simulink model "momentum_controller"  (R2020b)
settings: Solver=VariableStepAuto  StartTime=0.0  StopTime=100  RelTol=1e-3
values from neighbouring files (symbols this model uses):
  J = 0.001    [PMSM_params.m]
  Ls = 0.1    [PMSM_params.m]
  Lsd = Ls    (= 0.1)    [PMSM_params.m]
  Lsq = Ls    (= 0.1)    [PMSM_params.m]
  psi_f = 1    [PMSM_params.m]
  Rs = 10    [PMSM_params.m]
  Z = 1    [PMSM_params.m]
libraries: pid_lib x2
settings Model: Creator=Алексей  LastModifiedBy=Алексей

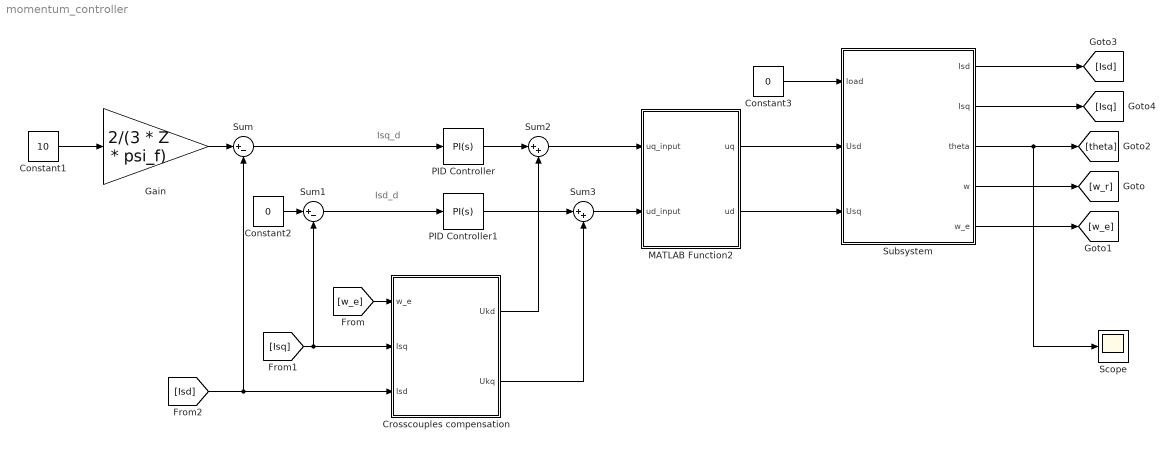
== system momentum_controller ==
  note: Isd_d
  note: Isq_d
  Constant1 : Constant  Value=10
  Constant2 : Constant  Value=0
  Constant3 : Constant  Value=0
  Crosscouples compensation : Subsystem
  Gain : Gain  Gain=2/(3 * Z * psi_f)
  MATLAB Function2 : MATLAB Function  TreatAsAtomicUnit=on
  PID Controller : pid_lib/PID Controller  Controller=PI  Form=Parallel  TimeDomain=Continuous-time  UseExternalTs=off  SampleTime=-1  IntegratorMethod=Forward Euler  FilterMethod=Forward Euler  ControllerParametersSource=internal  P=1  I=1  D=0  UseFilter=on  N=100  TunerSelectOption=Transfer Function Based (PID Tuner App)  InitialConditionSource=internal  InitialConditionForIntegrator=0  InitialConditionForFilter=0  DifferentiatorICPrevScaledInput=0  ExternalReset=none  TrackingMode=off  Kt=1  LimitOutput=off  SatLimitsSource=internal  UpperSaturationLimit=inf  LowerSaturationLimit=-inf  LinearizeAsGain=on  AntiWindupMode=none  Kb=1  POutMin=[]  POutMax=[]  IOutMin=[]  IOutMax=[]  DOutMin=[]  DOutMax=[]  NOutMin=[]  NOutMax=[]  SumOutMin=[]  SumOutMax=[]  SaturationOutMin=[]  SaturationOutMax=[]  PParamMin=[]  PParamMax=[]  IParamMin=[]  IParamMax=[]  DParamMin=[]  DParamMax=[]  NParamMin=[]  NParamMax=[]  KbParamMin=[]  KbParamMax=[]  KtParamMin=[]  KtParamMax=[]  KbOutMin=[]  KbOutMax=[]  KtOutMin=[]  KtOutMax=[]  IntegratorOutMin=[]  IntegratorOutMax=[]  FilterOutMin=[]  FilterOutMax=[]  SumI1OutMin=[]  SumI1OutMax=[]  SumI2OutMin=[]  SumI2OutMax=[]  SumI3OutMin=[]  SumI3OutMax=[]  SumI4OutMin=[]  SumI4OutMax=[]  SumDOutMin=[]  SumDOutMax=[]  DifferentiatorOutMin=[]  DifferentiatorOutMax=[]  FilterDiffOutCoefMin=[]  FilterDiffOutCoefMax=[]  ReciprocalOutMin=[]  ReciprocalOutMax=[]  SumDenOutMin=[]  SumDenOutMax=[]  SumNumOutMin=[]  SumNumOutMax=[]  DivideOutMin=[]  DivideOutMax=[]  UdiffTsProdOutMin=[]  UdiffTsProdOutMax=[]  NTsProdOutMin=[]  NTsProdOutMax=[]  UintegralTsProdOutMin=[]  UintegralTsProdOutMax=[]  UngainTsProdOutMin=[]  UngainTsProdOutMax=[]  IntegratorContinuousStateAttributes=''  IntegratorStateMustResolveToSignalObject=off  IntegratorRTWStateStorageClass=Auto  FilterContinuousStateAttributes=''  FilterStateMustResolveToSignalObject=off  FilterRTWStateStorageClass=Auto  ParallelPVariant=InternalParameters  IdealPVariant=Disabled  IVariant=InternalParameters  DVariant=Disabled  IntegratorVariant=Continuous  SatVariant=Disabled  AWVariant=Passthrough  PCopyVariant=Disabled  TRVariant=Disabled  FdbkBlocksVariant=Forward  IdealPFdbkVariant=Disabled  SatFdbkVariant=Disabled  DerivativeFilterVariant=Disabled  NVariant=Disabled  NCopyVariant=Disabled_SignalSpec  FilterICVariant=Disabled  IntegratorICVariant=InternalICs  ExternalResetVariant=Disabled  TRSumVariant=Passthrough  SumFdbkVariant=Disabled  SumVariant=Sum_PI  TsampFilterVariant=InternalTs  TsampNgainVariant=Passthrough  TsampIntegralVariant=Passthrough  ExternalSaturationOutDataTypeStr=Inherit: Same as second input
  PID Controller1 : pid_lib/PID Controller  Controller=PI  Form=Parallel  TimeDomain=Continuous-time  UseExternalTs=off  SampleTime=-1  IntegratorMethod=Forward Euler  FilterMethod=Forward Euler  ControllerParametersSource=internal  P=1  I=1  D=0  UseFilter=on  N=100  TunerSelectOption=Transfer Function Based (PID Tuner App)  InitialConditionSource=internal  InitialConditionForIntegrator=0  InitialConditionForFilter=0  DifferentiatorICPrevScaledInput=0  ExternalReset=none  TrackingMode=off  Kt=1  LimitOutput=off  SatLimitsSource=internal  UpperSaturationLimit=inf  LowerSaturationLimit=-inf  LinearizeAsGain=on  AntiWindupMode=none  Kb=1  POutMin=[]  POutMax=[]  IOutMin=[]  IOutMax=[]  DOutMin=[]  DOutMax=[]  NOutMin=[]  NOutMax=[]  SumOutMin=[]  SumOutMax=[]  SaturationOutMin=[]  SaturationOutMax=[]  PParamMin=[]  PParamMax=[]  IParamMin=[]  IParamMax=[]  DParamMin=[]  DParamMax=[]  NParamMin=[]  NParamMax=[]  KbParamMin=[]  KbParamMax=[]  KtParamMin=[]  KtParamMax=[]  KbOutMin=[]  KbOutMax=[]  KtOutMin=[]  KtOutMax=[]  IntegratorOutMin=[]  IntegratorOutMax=[]  FilterOutMin=[]  FilterOutMax=[]  SumI1OutMin=[]  SumI1OutMax=[]  SumI2OutMin=[]  SumI2OutMax=[]  SumI3OutMin=[]  SumI3OutMax=[]  SumI4OutMin=[]  SumI4OutMax=[]  SumDOutMin=[]  SumDOutMax=[]  DifferentiatorOutMin=[]  DifferentiatorOutMax=[]  FilterDiffOutCoefMin=[]  FilterDiffOutCoefMax=[]  ReciprocalOutMin=[]  ReciprocalOutMax=[]  SumDenOutMin=[]  SumDenOutMax=[]  SumNumOutMin=[]  SumNumOutMax=[]  DivideOutMin=[]  DivideOutMax=[]  UdiffTsProdOutMin=[]  UdiffTsProdOutMax=[]  NTsProdOutMin=[]  NTsProdOutMax=[]  UintegralTsProdOutMin=[]  UintegralTsProdOutMax=[]  UngainTsProdOutMin=[]  UngainTsProdOutMax=[]  IntegratorContinuousStateAttributes=''  IntegratorStateMustResolveToSignalObject=off  IntegratorRTWStateStorageClass=Auto  FilterContinuousStateAttributes=''  FilterStateMustResolveToSignalObject=off  FilterRTWStateStorageClass=Auto  ParallelPVariant=InternalParameters  IdealPVariant=Disabled  IVariant=InternalParameters  DVariant=Disabled  IntegratorVariant=Continuous  SatVariant=Disabled  AWVariant=Passthrough  PCopyVariant=Disabled  TRVariant=Disabled  FdbkBlocksVariant=Forward  IdealPFdbkVariant=Disabled  SatFdbkVariant=Disabled  DerivativeFilterVariant=Disabled  NVariant=Disabled  NCopyVariant=Disabled_SignalSpec  FilterICVariant=Disabled  IntegratorICVariant=InternalICs  ExternalResetVariant=Disabled  TRSumVariant=Passthrough  SumFdbkVariant=Disabled  SumVariant=Sum_PI  TsampFilterVariant=InternalTs  TsampNgainVariant=Passthrough  TsampIntegralVariant=Passthrough  ExternalSaturationOutDataTypeStr=Inherit: Same as second input
  Scope : Scope
  Subsystem : Subsystem
  Sum : Sum  Inputs=|+-
  Sum1 : Sum  Inputs=|+-
  Sum2 : Sum  Inputs=|++
  Sum3 : Sum  Inputs=|++
  wires:
  Constant1/1 -> Gain/1
  Gain/1 -> Sum/1
  Sum/1 -> PID Controller/1
  Constant2/1 -> Sum1/1
  Sum1/1 -> PID Controller1/1
  Constant3/1 -> Subsystem/1(load)
  Subsystem/3(theta) -> Scope/1, [theta]
  Subsystem/4(w) -> [w_r]
  Subsystem/5(w_e) -> [w_e]
  Subsystem/2(Isq) -> [Isq]
  Subsystem/1(Isd) -> [Isd]
  [w_e] -> Crosscouples compensation/1(w_e)
  [Isq] -> Sum1/2, Crosscouples compensation/2(Isq)
  [Isd] -> Crosscouples compensation/3(Isd), Sum/2
  PID Controller1/1 -> Sum3/1
  PID Controller/1 -> Sum2/1
  Crosscouples compensation/1(Ukd) -> Sum2/2
  Crosscouples compensation/2(Ukq) -> Sum3/2
  MATLAB Function2/1(uq) -> Subsystem/2(Usd)
  MATLAB Function2/2(ud) -> Subsystem/3(Usq)
  Sum2/1 -> MATLAB Function2/1(uq_input)
  Sum3/1 -> MATLAB Function2/2(ud_input)

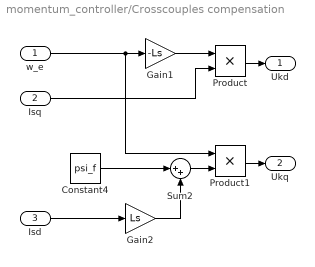
== system momentum_controller/Crosscouples compensation ==
  w_e : Inport
  Isq : Inport  Port=2
  Isd : Inport  Port=3
  Constant4 : Constant  Value=psi_f
  Gain1 : Gain  Gain=-Ls
  Gain2 : Gain  Gain=Ls
  Product : Product
  Product1 : Product
  Sum2 : Sum  Inputs=|++
  Ukd : Outport
  Ukq : Outport  Port=2
  wires:
  Isq/1 -> Product/2
  Gain2/1 -> Sum2/2
  w_e/1 -> Product1/1, Gain1/1
  Product/1 -> Ukd/1
  Constant4/1 -> Sum2/1
  Gain1/1 -> Product/1
  Product1/1 -> Ukq/1
  Isd/1 -> Gain2/1
  Sum2/1 -> Product1/2

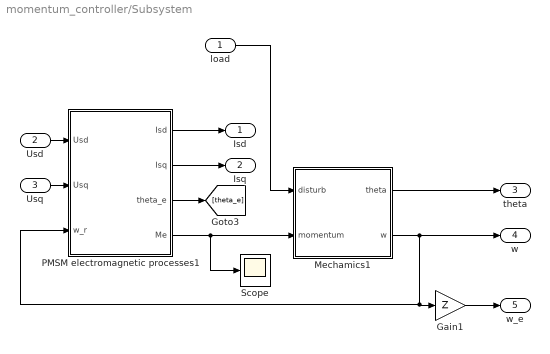
== system momentum_controller/Subsystem ==
  load : Inport
  Usd : Inport  Port=2
  Usq : Inport  Port=3
  Gain1 : Gain  Gain=Z
  Mechamics1 : Subsystem
  PMSM electromagnetic processes1 : Subsystem
  Scope : Scope
  Isd : Outport
  Isq : Outport  Port=2
  theta : Outport  Port=3
  w : Outport  Port=4
  w_e : Outport  Port=5
  wires:
  Mechamics1/2(w) -> w/1, PMSM electromagnetic processes1/3(w_r), Gain1/1
  PMSM electromagnetic processes1/3(theta_e) -> [theta_e]
  PMSM electromagnetic processes1/4(Me) -> Scope/1, Mechamics1/2(momentum)
  PMSM electromagnetic processes1/1(Isd) -> Isd/1
  Mechamics1/1(theta) -> theta/1
  Gain1/1 -> w_e/1
  load/1 -> Mechamics1/1(disturb)
  Usd/1 -> PMSM electromagnetic processes1/1(Usd)
  Usq/1 -> PMSM electromagnetic processes1/2(Usq)
  PMSM electromagnetic processes1/2(Isq) -> Isq/1

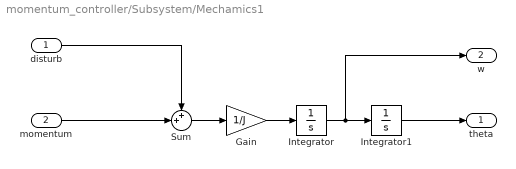
== system momentum_controller/Subsystem/Mechamics1 ==
  disturb : Inport
  momentum : Inport  Port=2
  Gain : Gain  Gain=1/J
  Integrator : Integrator
  Integrator1 : Integrator
  Sum : Sum  Inputs=++|
  theta : Outport  VectorParamsAs1DForOutWhenUnconnected=off
  w : Outport  Port=2  VectorParamsAs1DForOutWhenUnconnected=off
  wires:
  Gain/1 -> Integrator/1
  Sum/1 -> Gain/1
  Integrator1/1 -> theta/1
  momentum/1 -> Sum/2
  disturb/1 -> Sum/1
  Integrator/1 -> Integrator1/1, w/1

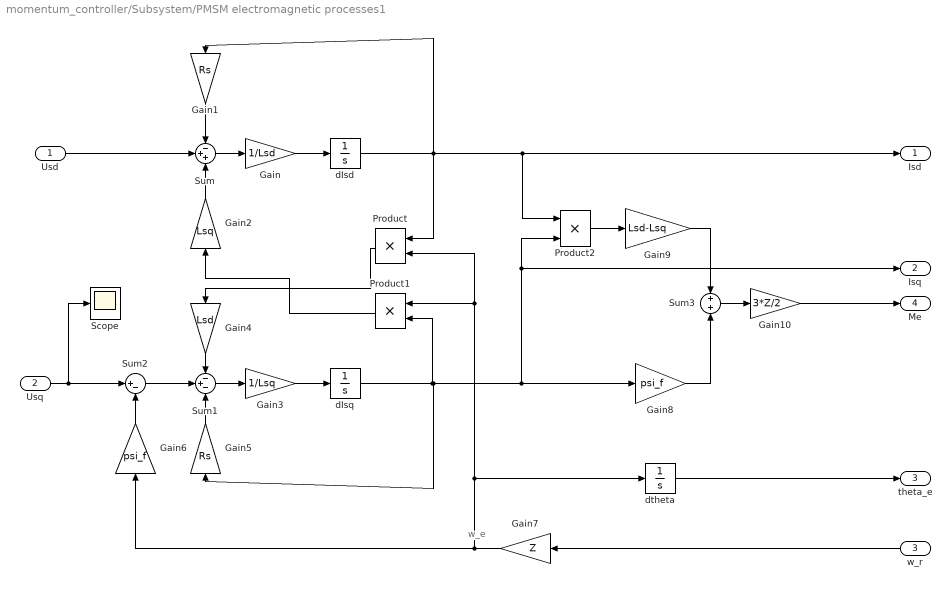
== system momentum_controller/Subsystem/PMSM electromagnetic processes1 ==
  note: w_e
  Usd : Inport
  Usq : Inport  Port=2
  w_r : Inport  Port=3
  Gain : Gain  Gain=1/Lsd
  Gain1 : Gain  Gain=Rs
  Gain10 : Gain  Gain=3*Z/2
  Gain2 : Gain  Gain=Lsq
  Gain3 : Gain  Gain=1/Lsq
  Gain4 : Gain  Gain=Lsd
  Gain5 : Gain  Gain=Rs
  Gain6 : Gain  Gain=psi_f
  Gain7 : Gain  Gain=Z
  Gain8 : Gain  Gain=psi_f
  Gain9 : Gain  Gain=Lsd-Lsq
  Product : Product
  Product1 : Product
  Product2 : Product
  Scope : Scope
  Sum : Sum  Inputs=-++
  Sum1 : Sum  Inputs=-+-
  Sum2 : Sum  Inputs=|+-
  Sum3 : Sum
  dIsd : Integrator
  dIsq : Integrator
  dtheta : Integrator
  Isd : Outport  VectorParamsAs1DForOutWhenUnconnected=off
  Isq : Outport  Port=2  VectorParamsAs1DForOutWhenUnconnected=off
  theta_e : Outport  Port=3  VectorParamsAs1DForOutWhenUnconnected=off
  Me : Outport  Port=4  VectorParamsAs1DForOutWhenUnconnected=off
  wires:
  Gain4/1 -> Sum1/1
  Sum2/1 -> Sum1/2
  Sum1/1 -> Gain3/1
  Gain3/1 -> dIsq/1
  Product/1 -> Gain4/1
  Gain6/1 -> Sum2/2
  Gain9/1 -> Sum3/1
  dIsq/1 -> Gain5/1, Isq/1, Product2/2, Gain8/1, Product1/2
  Gain2/1 -> Sum/3
  Sum/1 -> Gain/1
  Gain5/1 -> Sum1/3
  Sum3/1 -> Gain10/1
  Gain1/1 -> Sum/1
  Gain/1 -> dIsd/1
  dIsd/1 -> Gain1/1, Product/1, Product2/1, Isd/1
  Product1/1 -> Gain2/1
  Product2/1 -> Gain9/1
  Gain7/1 -> Gain6/1, Product/2, Product1/1, dtheta/1
  Gain8/1 -> Sum3/2
  Gain10/1 -> Me/1
  Usq/1 -> Scope/1, Sum2/1
  Usd/1 -> Sum/2
  w_r/1 -> Gain7/1
  dtheta/1 -> theta_e/1

== matlab function momentum_controller/MATLAB Function2 ==
  data: uq_input input; uq output; ud_input input; ud output; U_max parameter
function [uq, ud] = limit_U(uq_input, ud_input, U_max)
u_s_max = U_max / sqrt(3);
ud = U_max / sqrt(3);
uq = sqrt(u_s_max^2 - ud^2);
